simulink model "Zencar_rpo_2020_IDENTIFICATION_feedForwardModel_flywheelSpring"  (R2020a)
settings: Solver=VariableStepAuto  StartTime=0.0  StopTime=10.0  FixedStep=1e-3  RelTol=1e-3
values from neighbouring files (symbols this model uses):
  Asys = [0 1 0 ; -k/I -b/I cfi/I ; 0 -cfi/L -R/L]    [Zencar_rpo_2020_IDENTIFICATION_feedForwardScript_flywheelSpring.m]    (also in Zencar_rpo_2020_IDENTIFICATION_runScript_flywheelSpring.m; Zencar_rpo_2020_IDENTIFICATION_spesession_flywheelSpring.mat = [0  1  0; -6.68094218415  -0.797644539615  25.5045739424; 0 )
  Bsys = [0 ; 0 ; 1/L]    [Zencar_rpo_2020_IDENTIFICATION_feedForwardScript_flywheelSpring.m]    (also in Zencar_rpo_2020_IDENTIFICATION_runScript_flywheelSpring.m; Zencar_rpo_2020_IDENTIFICATION_spesession_flywheelSpring.mat = [0 0 166666.666667])
  cfi = cfi    [Zencar_rpo_2020_IDENTIFICATION_feedForwardScript_flywheelSpring.m]    (also in Zencar_rpo_2020_IDENTIFICATION_runScript_flywheelSpring.m; Zencar_rpo_2020_IDENTIFICATION_spesession_flywheelSpring.mat = 0.76328958575)
  Csys = [1 0 0;0 0 1]    [Zencar_rpo_2020_IDENTIFICATION_feedForwardScript_flywheelSpring.m]    (also in Zencar_rpo_2020_IDENTIFICATION_runScript_flywheelSpring.m; Zencar_rpo_2020_IDENTIFICATION_spesession_flywheelSpring.mat = [1  0  0; 0  0  1])
  Dsys = [0;0]    [Zencar_rpo_2020_IDENTIFICATION_feedForwardScript_flywheelSpring.m]    (also in Zencar_rpo_2020_IDENTIFICATION_runScript_flywheelSpring.m; Zencar_rpo_2020_IDENTIFICATION_spesession_flywheelSpring.mat = [0 0])
  fi_wanted = 2    [Zencar_rpo_2020_IDENTIFICATION_feedForwardScript_flywheelSpring.m]
  k = 0.312*ratio    [Zencar_rpo_2020_IDENTIFICATION_feedForwardScript_flywheelSpring.m]    (also in Zencar_rpo_2020_IDENTIFICATION_runScript_flywheelSpring.m; Zencar_rpo_2020_IDENTIFICATION_spesession_flywheelSpring.mat = 0.199944276806)
  R = 17.1102    [Zencar_rpo_2020_IDENTIFICATION_feedForwardScript_flywheelSpring.m]    (also in Zencar_rpo_2020_IDENTIFICATION_runScript_flywheelSpring.m; Zencar_rpo_2020_IDENTIFICATION_spesession_flywheelSpring.mat)
settings Model: Creator=Palo  LastModifiedBy=Palo

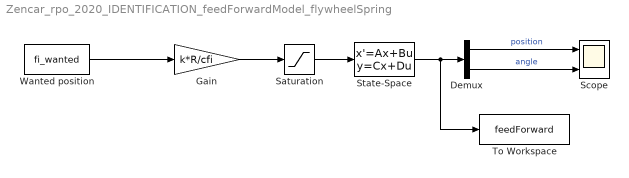
== system Zencar_rpo_2020_IDENTIFICATION_feedForwardModel_flywheelSpring ==
  Demux : Demux  Outputs=2
  Gain : Gain  Gain=k*R/cfi
  Saturation : Saturate  UpperLimit=12  LowerLimit=-12
  Scope : Scope  NumInputPorts=2
  State-Space : StateSpace  A=Asys  B=Bsys  C=Csys  D=Dsys  InitialCondition=0
  To Workspace : ToWorkspace  VariableName=feedForward  SaveFormat=Structure With Time  SampleTime=-1
  Wanted position : Constant  Value=fi_wanted
  wires:
  State-Space/1 -> To Workspace/1, Demux/1
  Demux/1 -> Scope/1  "position"
  Demux/2 -> Scope/2  "angle"
  Gain/1 -> Saturation/1
  Wanted position/1 -> Gain/1
  Saturation/1 -> State-Space/1
